simulink model "ChiefMaster_TTC580"  (R2022b)
settings: Solver=FixedStepAuto  StartTime=0.0  StopTime=10  FixedStep=0.01  RelTol=1e-3
values from neighbouring files (symbols this model uses):
  BattBox1_No = single(1)    [Parameters.m]
  BattBox2_No = single(2)    [Parameters.m]
  BattBox3_No = single(3)    [Parameters.m]
  CurrentLB = single(-3)    [Parameters.m]
  CurrentReductionConstant_Lvl0 = single(0.03)    [Parameters.m]
  CurrentReductionConstant_Lvl1 = single(0.05)    [Parameters.m]
  CurrentReductionConstant_Lvl2 = single(0.07)    [Parameters.m]
  CurrentReductionConstant_Lvl3 = single(0.1)    [Parameters.m]
  CurrentUB = single(3)    [Parameters.m]
  DCHV_Minus_In_Delay_ms = single(500)    [Parameters.m]
  FL_sHVC_CellBalanceVoltage_mV = single(3500)    [Parameters.m]
  FL_sInrushCurrent_dividebyzero = single(0.00001)    [Parameters.m]
  FL_u8HMI_BuzzerTimer = uint8(3)    [Parameters.m]
  IP_boActValue = true    [Parameters.m]
  IP_boDeactValue = false    [Parameters.m]
  IP_boInitValue = false    [Parameters.m]
  IP_s_LB = 18000    [Parameters.m]
  IP_s_UB = 22000    [Parameters.m]
  IP_sBatt1_ChargeCurrentMax_Factor = single(0.1)    [Parameters.m]
  IP_sBatt1_ChargeCurrentMax_LB = single(0)    [Parameters.m]
  IP_sBatt1_ChargeCurrentMax_Offset = single(0)    [Parameters.m]
  IP_sBatt1_ChargeCurrentMax_UB = single(6553.5)    [Parameters.m]
  IP_sBatt1_Current_Factor = single(0.1)    [Parameters.m]
  IP_sBatt1_Current_LB = single(-3276.8)    [Parameters.m]
  IP_sBatt1_Current_Offset = single(0)    [Parameters.m]
  IP_sBatt1_Current_UB = single(3276.8)    [Parameters.m]
  IP_sBatt1_DisChargeCurrentMax_Factor = single(0.1)    [Parameters.m]
  IP_sBatt1_DisChargeCurrentMax_LB = single(0)    [Parameters.m]
  IP_sBatt1_DisChargeCurrentMax_Offset = single(0)    [Parameters.m]
  IP_sBatt1_DisChargeCurrentMax_UB = single(6553.5)    [Parameters.m]
  IP_sBatt1_InsulationResistance_Factor = single(5)    [Parameters.m]
  IP_sBatt1_InsulationResistance_LB = single(0)    [Parameters.m]
  IP_sBatt1_InsulationResistance_Offset = single(0)    [Parameters.m]
  IP_sBatt1_InsulationResistance_UB = single(0)    [Parameters.m]
  IP_sBatt1_LiBa_IntResist_mOhm = single(25)    [Parameters.m]
  IP_sBatt1_SOC_Factor = single(1)    [Parameters.m]
  IP_sBatt1_SOC_LB = single(0)    [Parameters.m]
  IP_sBatt1_SOC_Offset = single(0)    [Parameters.m]
  IP_sBatt1_SOC_UB = single(100)    [Parameters.m]
  IP_sBatt1_SOH_Factor = single(1)    [Parameters.m]
  IP_sBatt1_SOH_LB = single(0)    [Parameters.m]
  IP_sBatt1_SOH_Offset = single(0)    [Parameters.m]
  IP_sBatt1_SOH_UB = single(100)    [Parameters.m]
  IP_sBatt1_Ubatt_Factor = single(0.1)    [Parameters.m]
  IP_sBatt1_Ubatt_LB = single(0)    [Parameters.m]
  IP_sBatt1_Ubatt_Offset = single(0)    [Parameters.m]
  IP_sBatt1_Ubatt_UB = single(6553.5)    [Parameters.m]
  IP_sBatt1_UserRi_Factor = single(1)    [Parameters.m]
  IP_sBatt1_UserRi_LB = single(0)    [Parameters.m]
  IP_sBatt1_UserRi_Offset = single(0)    [Parameters.m]
  IP_sBatt1_UserRi_UB = single(255)    [Parameters.m]
  IP_sBatt1_VoltageAtSensor_Factor = single(0.02)    [Parameters.m]
  IP_sBatt1_VoltageAtSensor_LB = single(0)    [Parameters.m]
  IP_sBatt1_VoltageAtSensor_Offset = single(0)    [Parameters.m]
  IP_sBatt1_VoltageAtSensor_UB = single(1310.7)    [Parameters.m]
  IP_sBatt2_LiBa_IntResist_mOhm = single(25)    [Parameters.m]
  IP_sBatt3_LiBa_IntResist_mOhm = single(25)    [Parameters.m]
  IP_sEM_LB = 2000    [Parameters.m]
  IP_sEM_UB = 8000    [Parameters.m]
  IP_sFB_LB = 5000    [Parameters.m]
  IP_sFB_UB = 10000    [Parameters.m]
  IP_sHVIL_LB = 12000    [Parameters.m]
  IP_sHVIL_UB = 15000    [Parameters.m]
  IP_sLoad_Voltage_Factor = single(1)    [Parameters.m]
  IP_sLoad_Voltage_LB = single(0)    [Parameters.m]
  IP_sLoad_Voltage_Offset = single(0)    [Parameters.m]
  IP_sLoad_Voltage_UB = single(65535)    [Parameters.m]
  IP_u8HVIL_Delay_ms = uint8(100)    [Parameters.m]
  IP_u8HW_IN_delay_ms = uint8(100)    [Parameters.m]
  IT_sInsulationSafeValue_kOhm = single(650)    [Parameters.m]
  IT_u8IMD_DelayTime_s = uint8(20)    [Parameters.m]
  MainHV_Minus_In_Delay = single(5)    [Parameters.m]
  MainHV_StatusDelay = single(5)    [Parameters.m]
  NotAvailable_uint16 = single(65535)    [Parameters.m]
  NotAvailable_uint8 = uint8(255)    [Parameters.m]
  OP_boHVIL_Supply = boolean(1)    [Parameters.m]
  SafeCurrentToCloseHV_A = single(5)    [Parameters.m]
  SafeVoltageToCloseHV_V = single(0.5)    [Parameters.m]
  UnexpectedBattChargingFcn_Available = boolean(1)    [Parameters.m]
  Voltage_NA_UB = uint16(65535)    [Parameters.m]
  VoltageSensorAvailableBB1 = boolean(0)    [Parameters.m]
  VoltageSensorAvailableBB2 = boolean(0)    [Parameters.m]
  VoltageSensorAvailableBB3 = boolean(0)    [Parameters.m]
libraries: simulink x184, Library_DataProcessing_v1_1 x167, Library_DataProcessing_v1 x142, libCM x28
(part 8 of 19)

== system ChiefMaster_TTC580/ChiefMaster/Input Translation/Battery Signals/Subsystem9 ==
  IP_Databus : Inport
  Bus Selector1 : BusSelector  OutputSignals=IP_Actia_BatBox_DataBus.IP_Actia_Batt1_Databus.Batt1_MyStatus2_Databus.IP_boBatt1_HV_relay_MINUS_Sense,IP_LB_BattBox_DataBus.IP_LB_BattBox1_DataBus.IP_LB_Batt1_Status01_DataBus.IP_LB_BMS_IO_state_Input_DataBus,IP_Actia_BatBox_DataBus.IP_Actia_Batt1_Databus.Batt1_MyStatus2_Databus.IP_boBatt1_HV_relay_PLUS_Sense,IP_Actia_BatBox_DataBus.IP_Actia_Batt2_Databus.Batt2_MyStatus2_Databus.IP_boBatt2_HV_relay_MINUS_Sense,IP_LB_BattBox_DataBus.IP_LB_BattBox2_DataBus.IP_LB_Batt2_Status01_DataBus.IP_LB_BMS_IO_state_Input_DataBus,IP_Actia_BatBox_DataBus.IP_Actia_Batt2_Databus.Batt2_MyStatus2_Databus.IP_boBatt2_HV_relay_PLUS_Sense,IP_Actia_BatBox_DataBus.IP_Actia_Batt3_Databus.Batt3_MyStatus2_Databus.IP_boBatt3_HV_relay_MINUS_Sense,IP_LB_BattBox_DataBus.IP_LB_BattBox3_DataBus.IP_LB_Batt3_Status01_DataBus.IP_LB_BMS_IO_state_Input_DataBus,IP_Actia_BatBox_DataBus.IP_Actia_Batt3_Databus.Batt3_MyStatus2_Databus.IP_boBatt3_HV_relay_PLUS_Sense
  Subsystem1 : Subsystem
  Subsystem2 : Subsystem
  Subsystem3 : Subsystem
  Subsystem4 : Subsystem
  Subsystem5 : Subsystem
  Subsystem8 : Subsystem
  IP_boBMS_HV_Minus_Sense_BB1 : Outport
  IP_boBMS_HV_Plus_Sense_BB1 : Outport  Port=2
  IP_boBMS_HV_Minus_Sense_BB2 : Outport  Port=3
  IP_boBMS_HV_Plus_Sense_BB2 : Outport  Port=4
  IP_boBMS_HV_Minus_Sense_BB3 : Outport  Port=5
  IP_boBMS_HV_Plus_Sense_BB3 : Outport  Port=6
  wires:
  Bus Selector1/6 -> Subsystem2/2(<IP_boBatt1_HV_relay_PLUS_Sense>)  "<IP_boBatt2_HV_relay_PLUS_Sense>"
  Bus Selector1/2 -> Subsystem8/2(<IP_LB_BMS_IO_state_Input_DataBus>), Subsystem1/1(<IP_LB_BMS_IO_state_Input_DataBus>)  "<IP_LB_BMS_IO_state_Input_DataBus>"
  Bus Selector1/5 -> Subsystem3/2(<IP_LB_BMS_IO_state_Input_DataBus>), Subsystem2/1(<IP_LB_BMS_IO_state_Input_DataBus>)  "<IP_LB_BMS_IO_state_Input_DataBus>"
  Bus Selector1/7 -> Subsystem5/1(<IP_boBatt3_HV_relay_MINUS_Sense>)  "<IP_boBatt3_HV_relay_MINUS_Sense>"
  Bus Selector1/9 -> Subsystem4/2(<IP_boBatt3_HV_relay_PLUS_Sense>)  "<IP_boBatt3_HV_relay_PLUS_Sense>"
  Bus Selector1/8 -> Subsystem5/2(<IP_LB_BMS_IO_state_Input_DataBus>), Subsystem4/1(<IP_LB_BMS_IO_state_Input_DataBus>)  "<IP_LB_BMS_IO_state_Input_DataBus>"
  Subsystem8/1(IP_boBMS_HV_Minus_Sense_BB1) -> IP_boBMS_HV_Minus_Sense_BB1/1
  IP_Databus/1 -> Bus Selector1/1
  Subsystem1/1(IP_boBMS_HV_Plus_Sense_BB1) -> IP_boBMS_HV_Plus_Sense_BB1/1
  Bus Selector1/4 -> Subsystem3/1(<IP_boBatt2_HV_relay_MINUS_Sense>)  "<IP_boBatt2_HV_relay_MINUS_Sense>"
  Subsystem2/1(IP_boBMS_HV_Plus_Sense_BB2) -> IP_boBMS_HV_Plus_Sense_BB2/1
  Subsystem3/1(IP_boBMS_HV_Minus_Sense_BB2) -> IP_boBMS_HV_Minus_Sense_BB2/1
  Subsystem5/1(IP_boBMS_HV_Minus_Sense_BB3) -> IP_boBMS_HV_Minus_Sense_BB3/1
  Subsystem4/1(IP_boBMS_HV_Plus_Sense_BB3) -> IP_boBMS_HV_Plus_Sense_BB3/1
  Bus Selector1/3 -> Subsystem1/2(<IP_boBatt1_HV_relay_PLUS_Sense>)  "<IP_boBatt1_HV_relay_PLUS_Sense>"
  Bus Selector1/1 -> Subsystem8/1(<IP_boBatt1_HV_relay_MINUS_Sense>)  "<IP_boBatt1_HV_relay_MINUS_Sense>"

== system ChiefMaster_TTC580/ChiefMaster/Output Processing/CM_OBD/CM_BDU_Msg5_6 ==
  OT_Databus : Inport
  Bus Selector1 : BusSelector  OutputSignals=OT_BDUControl_Databus.OT_boREQ_MainHV_ON_MINUS,OT_BDUControl_Databus.OT_boREQ_MainHV_ON_Precharge,OT_BDUControl_Databus.OT_boREQ_MainHV_ON_PLUS,OT_BDUControl_Databus.OT_boMainHV_Minus_Welded,OT_BDUControl_Databus.OT_boMainHV_Plus_Welded,OT_BDUControl_Databus.OT_boMainHV_WeldingCheckActive,OT_BDUControl_Databus.OT_u8MainHV_Minus_Status,OT_BDUControl_Databus.OT_u8MainHV_Plus_Status,OT_BDUControl_Databus.OT_u8Precharge_Status,OT_BDUControl_Databus.OT_u8WeldingDetection_Status,OT_BDUControl_Databus.OT_u8DCHV_Minus_Status,OT_BDUControl_Databus.OT_u8DCHV_plus_Status
  Bus Selector9 : BusSelector  OutputSignals=FL_Databus.FL_BatteryBox_HVControl_Databus.FL_sCalculated_VoltageDiff_BB1,FL_Databus.FL_BatteryBox_HVControl_Databus.FL_sCalculated_VoltageDiff_BB2,FL_Databus.FL_BatteryBox_HVControl_Databus.FL_sCalculated_VoltageDiff_BB3,FL_Databus.FL_BatteryBox_HVControl_Databus.FL_sCalculated_InrushCurrent_BB1,FL_Databus.FL_BatteryBox_HVControl_Databus.FL_sCalculated_InrushCurrent_BB2,FL_Databus.FL_BatteryBox_HVControl_Databus.FL_sCalculated_InrushCurrent_BB3
  Constant : Constant  Value=0  OutDataTypeStr=uint8
  Constant1 : Constant  Value=0  OutDataTypeStr=uint8
  Constant2 : Constant  Value=0  OutDataTypeStr=uint8
  Extract Bits{1..6} (6 alike) : simulink/Logic and Bit Operations/Extract Bits  bitsToExtract=Range of bits  numBits=8  bitIdxRange=[0 1]  outScalingMode=Preserve fixed-point scaling
  Lib_MultiBit_Concat1 : Library_DataProcessing_v1/Lib_MultiBit_Concat  SystemSampleTime=-1  VariantActivationTime=update diagram  Latency=0  AutoFrameSizeCalculation=off
  Lib_MultiBit_Concat2 : Library_DataProcessing_v1/Lib_MultiBit_Concat  SystemSampleTime=-1  VariantActivationTime=update diagram  Latency=0  AutoFrameSizeCalculation=off
  Lib_MultiBit_Concat7 : Library_DataProcessing_v1/Lib_MultiBit_Concat  SystemSampleTime=-1  VariantActivationTime=update diagram  Latency=0  AutoFrameSizeCalculation=off
  Mux3 : Mux  Inputs=8
  Mux4 : Mux  Inputs=8
  Subsystem1 : Subsystem
  Subsystem4 : Subsystem
  Subsystem5 : Subsystem
  Subsystem6 : Subsystem
  Subsystem8 : Subsystem
  Subsystem9 : Subsystem
  "Chief_Master_Calc_Msg5 " : Outport
  Chief_Master_BDU_Msg6 : Outport  Port=2
  wires:
  Extract Bits4/1 -> Lib_MultiBit_Concat1/5
  Bus Selector1/3 -> Lib_MultiBit_Concat7/3  "<OT_boREQ_MainHV_ON_PLUS>"
  Lib_MultiBit_Concat1/1 -> Mux4/6
  Constant/1 -> Lib_MultiBit_Concat1/8, Lib_MultiBit_Concat1/2, Lib_MultiBit_Concat7/8, Lib_MultiBit_Concat1/4, Lib_MultiBit_Concat1/6, Lib_MultiBit_Concat1/7
  Bus Selector9/1 -> Subsystem4/1(Calculated_VtgDiff_BB1)  "<FL_sCalculated_VoltageDiff_BB1>"
  Extract Bits2/1 -> Lib_MultiBit_Concat7/7
  Subsystem4/2(u8byte_MSB) -> Mux3/2
  Subsystem6/2(u8byte_MSB) -> Mux3/6
  Bus Selector1/5 -> Lib_MultiBit_Concat7/5  "<OT_boMainHV_Plus_Welded>"
  Bus Selector1/10 -> Extract Bits4/1  "<OT_u8WeldingDetection_Status>"
  Bus Selector1/8 -> Extract Bits1/1  "<OT_u8MainHV_Plus_Status>"
  Extract Bits3/1 -> Lib_MultiBit_Concat1/3
  Subsystem5/2(u8byte_MSB) -> Mux3/4
  Lib_MultiBit_Concat7/1 -> Mux4/5
  Subsystem4/1(u8byte_LSB) -> Mux3/1
  Subsystem9/2(u8byte_MSB) -> Mux4/4
  Subsystem1/1(u8byte_LSB) -> Mux3/7
  Subsystem5/1(u8byte_LSB) -> Mux3/3
  Subsystem9/1(u8byte_LSB) -> Mux4/3
  Subsystem6/1(u8byte_LSB) -> Mux3/5
  Bus Selector9/2 -> Subsystem5/1(Calculated_VtgDiff_BB2)  "<FL_sCalculated_VoltageDiff_BB2>"
  Bus Selector9/5 -> Subsystem8/1(Calculated_InrushCurr_BB2)  "<FL_sCalculated_InrushCurrent_BB2>"
  Bus Selector9/3 -> Subsystem6/1(Calculated_VtgDiff_BB3)  "<FL_sCalculated_VoltageDiff_BB3>"
  Bus Selector1/4 -> Lib_MultiBit_Concat7/4  "<OT_boMainHV_Minus_Welded>"
  Bus Selector9/4 -> Subsystem1/1(Calculated_InrushCurr_BB2)  "<FL_sCalculated_InrushCurrent_BB1>"
  Bus Selector9/6 -> Subsystem9/1(Calculated_InrushCurr_BB3)  "<FL_sCalculated_InrushCurrent_BB3>"
  Bus Selector1/7 -> Extract Bits2/1  "<OT_u8MainHV_Minus_Status>"
  Bus Selector1/1 -> Lib_MultiBit_Concat7/1  "<OT_boREQ_MainHV_ON_MINUS>"
  Subsystem8/2(u8byte_MSB) -> Mux4/2
  Bus Selector1/9 -> Extract Bits3/1  "<OT_u8Precharge_Status>"
  Constant1/1 -> Mux4/8
  Mux4/1 -> Chief_Master_BDU_Msg6/1
  Mux3/1 -> "Chief_Master_Calc_Msg5 "/1
  Subsystem8/1(u8byte_LSB) -> Mux4/1
  Bus Selector1/2 -> Lib_MultiBit_Concat7/2  "<OT_boREQ_MainHV_ON_Precharge>"
  OT_Databus/1 -> Bus Selector1/1, Bus Selector9/1
  Subsystem1/2(u8byte_MSB) -> Mux3/8
  Bus Selector1/6 -> Lib_MultiBit_Concat7/6  "<OT_boMainHV_WeldingCheckActive>"
  Extract Bits1/1 -> Lib_MultiBit_Concat1/1
  Constant2/1 -> Lib_MultiBit_Concat2/8, Lib_MultiBit_Concat2/7, Lib_MultiBit_Concat2/6, Lib_MultiBit_Concat2/5, Lib_MultiBit_Concat2/4, Lib_MultiBit_Concat2/2
  Lib_MultiBit_Concat2/1 -> Mux4/7
  Bus Selector1/11 -> Extract Bits5/1  "<OT_u8DCHV_Minus_Status>"
  Extract Bits5/1 -> Lib_MultiBit_Concat2/1
  Extract Bits6/1 -> Lib_MultiBit_Concat2/3
  Bus Selector1/12 -> Extract Bits6/1  "<OT_u8DCHV_plus_Status>"

== system ChiefMaster_TTC580/ChiefMaster/Output Processing/CM_OBD/CM_Battery1_Msg7 ==
  OT_Databus : Inport
  Bus Selector1 : BusSelector  OutputSignals=FL_Databus.IT_Databus.IT_BatterySignal_Databus.IT_sBMS_VtgInt_BB1,FL_Databus.IT_Databus.IT_BatterySignal_Databus.IT_sBMS_Current_BB1,FL_Databus.IT_Databus.IT_BatterySignal_Databus.IT_u8BMS_SOC_BB1,FL_Databus.IT_Databus.IT_BatterySignal_Databus.IT_sBMS_InternalResistance_BB1_ohms
  Bus Selector2 : BusSelector  OutputSignals=FL_Databus.IT_Databus.IT_BatterySignal_Databus.IT_boBMS_HV_REL_ON_BB1,FL_Databus.IT_Databus.IT_BatterySignal_Databus.IT_boBMS_HV_Minus_Sense_BB1,FL_Databus.IT_Databus.IT_BatterySignal_Databus.IT_boBMS_HV_Plus_Sense_BB1,FL_Databus.IT_Databus.IT_BatterySignal_Databus.IT_boBMS_InsulationReadyOK_B1,FL_Databus.IT_Databus.IT_BatterySignal_Databus.IT_boBMS_InsulationSDError_B1,FL_Databus.IT_Databus.IT_BatterySignal_Databus.IT_boBMS_IMD_Active_BB1,FL_Databus.IT_Databus.IT_BatterySignal_Databus.IT_boBMS_Error_BB1,FL_Databus.IT_Databus.IT_BatterySignal_Databus.IT_boBMS_Warning_BB1
  Bus Selector6 : BusSelector  OutputSignals=FL_Databus.IT_Databus.IT_BatterySignal_Databus.IT_boBMS_Batt1_Availability,OT_IMD_Databus.OT_boREQ_IMD_ON_BB1,OT_BatteryBox_HVControl_Databus.OT_u8ContactorState_BB1,OT_BatteryBox_HVControl_Databus.OT_boREQ_HV_ON_BB1,OT_BatteryBox_HVControl_Databus.OT_u8Contactor_FB_State_BB1,FL_Databus.IT_Databus.IT_BatterySignal_Databus.IT_boBMS_SDError_BB1
  Constant : Constant  Value=0  OutDataTypeStr=single
  Constant1 : Constant  Value=0  OutDataTypeStr=single
  Constant2 : Constant  Value=0.1  OutDataTypeStr=single
  Constant3 : Constant  Value=0.1  OutDataTypeStr=single
  Constant4 : Constant  Value=0  OutDataTypeStr=uint8
  Data Type Conversion1 : DataTypeConversion  OutDataTypeStr=uint8  SaturateOnIntegerOverflow=off  RndMeth=Floor
  Extract Bits1 : simulink/Logic and Bit Operations/Extract Bits  bitsToExtract=Range of bits  numBits=8  bitIdxRange=[0 1]  outScalingMode=Preserve fixed-point scaling
  Extract Bits2 : simulink/Logic and Bit Operations/Extract Bits  bitsToExtract=Range of bits  numBits=8  bitIdxRange=[0 1]  outScalingMode=Preserve fixed-point scaling
  Lib_2bytes_Split1 : Library_DataProcessing_v1/Lib_2bytes_Split  SystemSampleTime=-1  VariantActivationTime=update diagram  Latency=0  AutoFrameSizeCalculation=off
  Lib_2bytes_Split2 : Library_DataProcessing_v1/Lib_2bytes_Split  SystemSampleTime=-1  VariantActivationTime=update diagram  Latency=0  AutoFrameSizeCalculation=off
  Lib_MultiBit_Concat1 : Library_DataProcessing_v1/Lib_MultiBit_Concat  SystemSampleTime=-1  VariantActivationTime=update diagram  Latency=0  AutoFrameSizeCalculation=off
  Lib_MultiBit_Concat2 : Library_DataProcessing_v1/Lib_MultiBit_Concat  SystemSampleTime=-1  VariantActivationTime=update diagram  Latency=0  AutoFrameSizeCalculation=off
  Lib_OutProcessing1 : Library_DataProcessing_v1/Lib_OutProcessing  SystemSampleTime=-1  VariantActivationTime=update diagram  Latency=0  AutoFrameSizeCalculation=off
  Lib_OutProcessing2 : Library_DataProcessing_v1/Lib_OutProcessing  SystemSampleTime=-1  VariantActivationTime=update diagram  Latency=0  AutoFrameSizeCalculation=off
  Mux : Mux  Inputs=8
  OP_ChiefMaster_Battery1_Msg7 : Outport
  wires:
  Mux/1 -> OP_ChiefMaster_Battery1_Msg7/1
  OT_Databus/1 -> Bus Selector1/1, Bus Selector2/1, Bus Selector6/1
  Bus Selector6/1 -> Lib_MultiBit_Concat1/1  "<IT_boBMS_Batt1_Availability>"
  Bus Selector6/2 -> Lib_MultiBit_Concat1/2  "<OT_boREQ_IMD_ON_BB1>"
  Bus Selector6/3 -> Extract Bits2/1  "<OT_u8ContactorState_BB1>"
  Bus Selector6/4 -> Lib_MultiBit_Concat1/5  "<OT_boREQ_HV_ON_BB1>"
  Bus Selector6/5 -> Extract Bits1/1  "<OT_u8Contactor_FB_State_BB1>"
  Lib_MultiBit_Concat1/1 -> Mux/1
  Lib_MultiBit_Concat2/1 -> Mux/2
  Constant/1 -> Lib_OutProcessing1/2
  Constant2/1 -> Lib_OutProcessing1/3
  Lib_OutProcessing1/1 -> Lib_2bytes_Split1/1
  Bus Selector1/1 -> Lib_OutProcessing1/1  "<IT_sBMS_VtgInt_BB1>"
  Lib_2bytes_Split1/1 -> Mux/3
  Lib_2bytes_Split1/2 -> Mux/4
  Bus Selector1/2 -> Lib_OutProcessing2/1  "<IT_sBMS_Current_BB1>"
  Lib_OutProcessing2/1 -> Lib_2bytes_Split2/1
  Constant3/1 -> Lib_OutProcessing2/3
  Constant1/1 -> Lib_OutProcessing2/2
  Lib_2bytes_Split2/1 -> Mux/5
  Lib_2bytes_Split2/2 -> Mux/6
  Bus Selector1/3 -> Mux/7  "<IT_u8BMS_SOC_BB1>"
  Bus Selector1/4 -> Data Type Conversion1/1  "<IT_sBMS_InternalResistance_BB1_ohms>"
  Data Type Conversion1/1 -> Mux/8
  Constant4/1 -> Lib_MultiBit_Concat1/4, Lib_MultiBit_Concat1/7
  Extract Bits2/1 -> Lib_MultiBit_Concat1/3
  Extract Bits1/1 -> Lib_MultiBit_Concat1/6
  Bus Selector6/6 -> Lib_MultiBit_Concat1/8  "<IT_boBMS_SDError_BB1>"
  Bus Selector2/1 -> Lib_MultiBit_Concat2/1  "<IT_boBMS_HV_REL_ON_BB1>"
  Bus Selector2/2 -> Lib_MultiBit_Concat2/2  "<IT_boBMS_HV_Minus_Sense_BB1>"
  Bus Selector2/3 -> Lib_MultiBit_Concat2/3  "<IT_boBMS_HV_Plus_Sense_BB1>"
  Bus Selector2/4 -> Lib_MultiBit_Concat2/4  "<IT_boBMS_InsulationReadyOK_B1>"
  Bus Selector2/5 -> Lib_MultiBit_Concat2/5  "<IT_boBMS_InsulationSDError_B1>"
  Bus Selector2/6 -> Lib_MultiBit_Concat2/6  "<IT_boBMS_IMD_Active_BB1>"
  Bus Selector2/7 -> Lib_MultiBit_Concat2/7  "<IT_boBMS_Error_BB1>"
  Bus Selector2/8 -> Lib_MultiBit_Concat2/8  "<IT_boBMS_Warning_BB1>"

== system ChiefMaster_TTC580/ChiefMaster/Output Processing/CM_OBD/CM_Battery1_Msg8 ==
  OT_Databus : Inport
  Bus Selector1 : BusSelector  OutputSignals=FL_Databus.IT_Databus.IT_BatterySignal_Databus.IT_sBMS_ChargeCurrentPrognosis_BB1,FL_Databus.IT_Databus.IT_BatterySignal_Databus.IT_sBMS_DisChargeCurrentPrognosis_BB1,FL_Databus.IT_Databus.IT_BatterySignal_Databus.IT_sBMS_InsulationResistance_BB1,FL_Databus.IT_Databus.IT_BatterySignal_Databus.IT_boBMS_InsulationResistance_Minus_kOhm_BB1
  Constant{1..2,5,7} (4 alike) : Constant  Value=0  OutDataTypeStr=single
  Constant3 : Constant  Value=0.1  OutDataTypeStr=single
  Constant4 : Constant  Value=0.1  OutDataTypeStr=single
  Constant6 : Constant  Value=100  OutDataTypeStr=single
  Constant8 : Constant  Value=100  OutDataTypeStr=single
  Lib_2bytes_Split{1..4} (4 alike) : Library_DataProcessing_v1/Lib_2bytes_Split  SystemSampleTime=-1  VariantActivationTime=update diagram  Latency=0  AutoFrameSizeCalculation=off
  Lib_OutProcessing{1..4} (4 alike) : Library_DataProcessing_v1/Lib_OutProcessing  SystemSampleTime=-1  VariantActivationTime=update diagram  Latency=0  AutoFrameSizeCalculation=off
  Mux : Mux  Inputs=8
  OP_ChiefMaster_Battery1_Msg8 : Outport
  wires:
  OT_Databus/1 -> Bus Selector1/1
  Mux/1 -> OP_ChiefMaster_Battery1_Msg8/1
  Bus Selector1/1 -> Lib_OutProcessing2/1  "<IT_sBMS_ChargeCurrentPrognosis_BB1>"
  Bus Selector1/2 -> Lib_OutProcessing1/1  "<IT_sBMS_DisChargeCurrentPrognosis_BB1>"
  Bus Selector1/3 -> Lib_OutProcessing3/1  "<IT_sBMS_InsulationResistance_BB1>"
  Bus Selector1/4 -> Lib_OutProcessing4/1  "<IT_boBMS_InsulationResistance_Minus_kOhm_BB1>"
  Constant3/1 -> Lib_OutProcessing2/3
  Lib_OutProcessing2/1 -> Lib_2bytes_Split2/1
  Constant1/1 -> Lib_OutProcessing2/2
  Lib_2bytes_Split2/1 -> Mux/1
  Lib_2bytes_Split2/2 -> Mux/2
  Constant2/1 -> Lib_OutProcessing1/2
  Lib_OutProcessing1/1 -> Lib_2bytes_Split1/1
  Constant4/1 -> Lib_OutProcessing1/3
  Lib_2bytes_Split1/1 -> Mux/3
  Lib_2bytes_Split1/2 -> Mux/4
  Constant6/1 -> Lib_OutProcessing3/3
  Lib_OutProcessing3/1 -> Lib_2bytes_Split3/1
  Constant5/1 -> Lib_OutProcessing3/2
  Lib_2bytes_Split3/1 -> Mux/5
  Lib_2bytes_Split3/2 -> Mux/6
  Constant7/1 -> Lib_OutProcessing4/2
  Lib_OutProcessing4/1 -> Lib_2bytes_Split4/1
  Constant8/1 -> Lib_OutProcessing4/3
  Lib_2bytes_Split4/1 -> Mux/7
  Lib_2bytes_Split4/2 -> Mux/8

== system ChiefMaster_TTC580/ChiefMaster/Output Processing/CM_OBD/CM_Battery1_Msg9 ==
  OT_Databus : Inport
  Bus Selector1 : BusSelector  OutputSignals=FL_Databus.IT_Databus.IT_BatterySignal_Databus.IP_sBMS_MinTemp_degC_BB1,FL_Databus.IT_Databus.IT_BatterySignal_Databus.IP_sBMS_MaxTemp_degC_BB1,FL_Databus.IT_Databus.IT_BatterySignal_Databus.IP_sBMS_MinCellVoltage_BB1,FL_Databus.IT_Databus.IT_BatterySignal_Databus.IP_sBMS_MaxCellVoltage_BB1
  Constant1 : Constant  Value=-40  OutDataTypeStr=single
  Constant2 : Constant  Value=-40  OutDataTypeStr=single
  Constant3 : Constant  OutDataTypeStr=single
  Constant4 : Constant  OutDataTypeStr=single
  Constant5 : Constant  Value=0  OutDataTypeStr=single
  Constant6 : Constant  Value=0.1  OutDataTypeStr=single
  Constant7 : Constant  Value=0  OutDataTypeStr=single
  Constant8 : Constant  Value=0.1  OutDataTypeStr=single
  Constant9 : Constant  Value=0  OutDataTypeStr=uint8
  Data Type Conversion : DataTypeConversion  OutDataTypeStr=uint8  SaturateOnIntegerOverflow=off  RndMeth=Floor
  Data Type Conversion1 : DataTypeConversion  OutDataTypeStr=uint8  SaturateOnIntegerOverflow=off  RndMeth=Floor
  Lib_2bytes_Split3 : Library_DataProcessing_v1/Lib_2bytes_Split  SystemSampleTime=-1  VariantActivationTime=update diagram  Latency=0  AutoFrameSizeCalculation=off
  Lib_2bytes_Split4 : Library_DataProcessing_v1/Lib_2bytes_Split  SystemSampleTime=-1  VariantActivationTime=update diagram  Latency=0  AutoFrameSizeCalculation=off
  Lib_OutProcessing{1..4} (4 alike) : Library_DataProcessing_v1/Lib_OutProcessing  SystemSampleTime=-1  VariantActivationTime=update diagram  Latency=0  AutoFrameSizeCalculation=off
  Mux : Mux  Inputs=8
  OP_ChiefMaster_Battery1_Msg8 : Outport
  wires:
  Constant8/1 -> Lib_OutProcessing4/3
  Lib_OutProcessing4/1 -> Lib_2bytes_Split4/1
  Constant7/1 -> Lib_OutProcessing4/2
  Constant5/1 -> Lib_OutProcessing3/2
  Lib_OutProcessing3/1 -> Lib_2bytes_Split3/1
  Constant6/1 -> Lib_OutProcessing3/3
  Constant4/1 -> Lib_OutProcessing1/3
  Lib_OutProcessing1/1 -> Data Type Conversion1/1
  Constant2/1 -> Lib_OutProcessing1/2
  Constant1/1 -> Lib_OutProcessing2/2
  Lib_OutProcessing2/1 -> Data Type Conversion/1
  Constant3/1 -> Lib_OutProcessing2/3
  Bus Selector1/4 -> Lib_OutProcessing4/1  "<IP_sBMS_MaxCellVoltage_BB1>"
  Bus Selector1/3 -> Lib_OutProcessing3/1  "<IP_sBMS_MinCellVoltage_BB1>"
  Bus Selector1/2 -> Lib_OutProcessing1/1  "<IP_sBMS_MaxTemp_degC_BB1>"
  Bus Selector1/1 -> Lib_OutProcessing2/1  "<IP_sBMS_MinTemp_degC_BB1>"
  Mux/1 -> OP_ChiefMaster_Battery1_Msg8/1
  OT_Databus/1 -> Bus Selector1/1
  Constant9/1 -> Mux/7, Mux/8
  Lib_2bytes_Split3/1 -> Mux/3
  Lib_2bytes_Split3/2 -> Mux/4
  Lib_2bytes_Split4/1 -> Mux/5
  Lib_2bytes_Split4/2 -> Mux/6
  Data Type Conversion/1 -> Mux/1
  Data Type Conversion1/1 -> Mux/2

== system ChiefMaster_TTC580/ChiefMaster/Output Processing/CM_OBD/CM_Battery2_Msg10 ==
  OT_Databus : Inport
  Bus Selector1 : BusSelector  OutputSignals=FL_Databus.IT_Databus.IT_BatterySignal_Databus.IT_sBMS_VtgInt_BB2,FL_Databus.IT_Databus.IT_BatterySignal_Databus.IT_sBMS_Current_BB2,FL_Databus.IT_Databus.IT_BatterySignal_Databus.IT_u8BMS_SOC_BB2,FL_Databus.IT_Databus.IT_BatterySignal_Databus.IT_sBMS_InternalResistance_BB2_ohms
  Bus Selector2 : BusSelector  OutputSignals=FL_Databus.IT_Databus.IT_BatterySignal_Databus.IT_boBMS_HV_REL_ON_BB2,FL_Databus.IT_Databus.IT_BatterySignal_Databus.IT_boBMS_HV_Minus_Sense_BB2,FL_Databus.IT_Databus.IT_BatterySignal_Databus.IT_boBMS_HV_Plus_Sense_BB2,FL_Databus.IT_Databus.IT_BatterySignal_Databus.IT_boBMS_InsulationReadyOK_B2,FL_Databus.IT_Databus.IT_BatterySignal_Databus.IT_boBMS_InsulationSDError_B2,FL_Databus.IT_Databus.IT_BatterySignal_Databus.IT_boBMS_IMD_Active_BB2,FL_Databus.IT_Databus.IT_BatterySignal_Databus.IT_boBMS_Error_BB2,FL_Databus.IT_Databus.IT_BatterySignal_Databus.IT_boBMS_Warning_BB2
  Bus Selector6 : BusSelector  OutputSignals=FL_Databus.IT_Databus.IT_BatterySignal_Databus.IT_boBMS_Batt2_Availability,OT_IMD_Databus.OT_boREQ_IMD_ON_BB2,OT_BatteryBox_HVControl_Databus.OT_u8ContactorState_BB2,OT_BatteryBox_HVControl_Databus.OT_boREQ_HV_ON_BB2,OT_BatteryBox_HVControl_Databus.OT_u8Contactor_FB_State_BB2,FL_Databus.IT_Databus.IT_BatterySignal_Databus.IT_boBMS_SDError_BB2
  Constant : Constant  Value=0  OutDataTypeStr=single
  Constant1 : Constant  Value=0  OutDataTypeStr=single
  Constant2 : Constant  Value=0.1  OutDataTypeStr=single
  Constant3 : Constant  Value=0.1  OutDataTypeStr=single
  Constant4 : Constant  Value=0  OutDataTypeStr=uint8
  Data Type Conversion : DataTypeConversion  SaturateOnIntegerOverflow=off  RndMeth=Floor
  Extract Bits1 : simulink/Logic and Bit Operations/Extract Bits  bitsToExtract=Range of bits  numBits=8  bitIdxRange=[0 1]  outScalingMode=Preserve fixed-point scaling
  Extract Bits2 : simulink/Logic and Bit Operations/Extract Bits  bitsToExtract=Range of bits  numBits=8  bitIdxRange=[0 1]  outScalingMode=Preserve fixed-point scaling
  Lib_2bytes_Split1 : Library_DataProcessing_v1/Lib_2bytes_Split  SystemSampleTime=-1  VariantActivationTime=update diagram  Latency=0  AutoFrameSizeCalculation=off
  Lib_2bytes_Split2 : Library_DataProcessing_v1/Lib_2bytes_Split  SystemSampleTime=-1  VariantActivationTime=update diagram  Latency=0  AutoFrameSizeCalculation=off
  Lib_MultiBit_Concat1 : Library_DataProcessing_v1/Lib_MultiBit_Concat  SystemSampleTime=-1  VariantActivationTime=update diagram  Latency=0  AutoFrameSizeCalculation=off
  Lib_MultiBit_Concat2 : Library_DataProcessing_v1/Lib_MultiBit_Concat  SystemSampleTime=-1  VariantActivationTime=update diagram  Latency=0  AutoFrameSizeCalculation=off
  Lib_OutProcessing1 : Library_DataProcessing_v1/Lib_OutProcessing  SystemSampleTime=-1  VariantActivationTime=update diagram  Latency=0  AutoFrameSizeCalculation=off
  Lib_OutProcessing2 : Library_DataProcessing_v1/Lib_OutProcessing  SystemSampleTime=-1  VariantActivationTime=update diagram  Latency=0  AutoFrameSizeCalculation=off
  Mux : Mux  Inputs=8
  OP_ChiefMaster_Battery2_Msg9 : Outport
  wires:
  Bus Selector1/4 -> Data Type Conversion/1  "<IT_sBMS_InternalResistance_BB2_ohms>"
  Bus Selector1/3 -> Mux/7  "<IT_u8BMS_SOC_BB2>"
  Lib_2bytes_Split2/2 -> Mux/6
  Lib_2bytes_Split2/1 -> Mux/5
  Constant1/1 -> Lib_OutProcessing2/2
  Constant3/1 -> Lib_OutProcessing2/3
  Lib_OutProcessing2/1 -> Lib_2bytes_Split2/1
  Bus Selector1/2 -> Lib_OutProcessing2/1  "<IT_sBMS_Current_BB2>"
  Lib_2bytes_Split1/2 -> Mux/4
  Lib_2bytes_Split1/1 -> Mux/3
  Bus Selector1/1 -> Lib_OutProcessing1/1  "<IT_sBMS_VtgInt_BB2>"
  Lib_OutProcessing1/1 -> Lib_2bytes_Split1/1
  Constant2/1 -> Lib_OutProcessing1/3
  Constant/1 -> Lib_OutProcessing1/2
  Lib_MultiBit_Concat2/1 -> Mux/2
  Lib_MultiBit_Concat1/1 -> Mux/1
  Bus Selector6/6 -> Lib_MultiBit_Concat1/8  "<IT_boBMS_SDError_BB2>"
  Bus Selector6/5 -> Extract Bits1/1  "<OT_u8Contactor_FB_State_BB2>"
  Bus Selector6/4 -> Lib_MultiBit_Concat1/5  "<OT_boREQ_HV_ON_BB2>"
  Bus Selector6/3 -> Extract Bits2/1  "<OT_u8ContactorState_BB2>"
  Bus Selector6/2 -> Lib_MultiBit_Concat1/2  "<OT_boREQ_IMD_ON_BB2>"
  Bus Selector6/1 -> Lib_MultiBit_Concat1/1  "<IT_boBMS_Batt2_Availability>"
  OT_Databus/1 -> Bus Selector6/1, Bus Selector1/1, Bus Selector2/1
  Mux/1 -> OP_ChiefMaster_Battery2_Msg9/1
  Data Type Conversion/1 -> Mux/8
  Extract Bits1/1 -> Lib_MultiBit_Concat1/6
  Extract Bits2/1 -> Lib_MultiBit_Concat1/3
  Constant4/1 -> Lib_MultiBit_Concat1/4, Lib_MultiBit_Concat1/7
  Bus Selector2/1 -> Lib_MultiBit_Concat2/1  "<IT_boBMS_HV_REL_ON_BB2>"
  Bus Selector2/2 -> Lib_MultiBit_Concat2/2  "<IT_boBMS_HV_Minus_Sense_BB2>"
  Bus Selector2/3 -> Lib_MultiBit_Concat2/3  "<IT_boBMS_HV_Plus_Sense_BB2>"
  Bus Selector2/4 -> Lib_MultiBit_Concat2/4  "<IT_boBMS_InsulationReadyOK_B2>"
  Bus Selector2/5 -> Lib_MultiBit_Concat2/5  "<IT_boBMS_InsulationSDError_B2>"
  Bus Selector2/6 -> Lib_MultiBit_Concat2/6  "<IT_boBMS_IMD_Active_BB2>"
  Bus Selector2/7 -> Lib_MultiBit_Concat2/7  "<IT_boBMS_Error_BB2>"
  Bus Selector2/8 -> Lib_MultiBit_Concat2/8  "<IT_boBMS_Warning_BB2>"

== system ChiefMaster_TTC580/ChiefMaster/Output Processing/CM_OBD/CM_Battery2_Msg11 ==
  OT_Databus : Inport
  Bus Selector1 : BusSelector  OutputSignals=FL_Databus.IT_Databus.IT_BatterySignal_Databus.IT_sBMS_ChargeCurrentPrognosis_BB2,FL_Databus.IT_Databus.IT_BatterySignal_Databus.IT_sBMS_DisChargeCurrentPrognosis_BB2,FL_Databus.IT_Databus.IT_BatterySignal_Databus.IT_sBMS_InsulationResistance_BB2,FL_Databus.IT_Databus.IT_BatterySignal_Databus.IT_boBMS_InsulationResistance_Minus_kOhm_BB2
  Constant{1..2,5,7} (4 alike) : Constant  Value=0  OutDataTypeStr=single
  Constant3 : Constant  Value=0.1  OutDataTypeStr=single
  Constant4 : Constant  Value=0.1  OutDataTypeStr=single
  Constant6 : Constant  Value=100  OutDataTypeStr=single
  Constant8 : Constant  Value=100  OutDataTypeStr=single
  Lib_2bytes_Split{1..4} (4 alike) : Library_DataProcessing_v1/Lib_2bytes_Split  SystemSampleTime=-1  VariantActivationTime=update diagram  Latency=0  AutoFrameSizeCalculation=off
  Lib_OutProcessing{1..4} (4 alike) : Library_DataProcessing_v1/Lib_OutProcessing  SystemSampleTime=-1  VariantActivationTime=update diagram  Latency=0  AutoFrameSizeCalculation=off
  Mux : Mux  Inputs=8
  OP_ChiefMaster_Battery2_Msg10 : Outport
  wires:
  Lib_2bytes_Split4/2 -> Mux/8
  Lib_2bytes_Split4/1 -> Mux/7
  Constant8/1 -> Lib_OutProcessing4/3
  Lib_OutProcessing4/1 -> Lib_2bytes_Split4/1
  Constant7/1 -> Lib_OutProcessing4/2
  Lib_2bytes_Split3/2 -> Mux/6
  Lib_2bytes_Split3/1 -> Mux/5
  Constant5/1 -> Lib_OutProcessing3/2
  Lib_OutProcessing3/1 -> Lib_2bytes_Split3/1
  Constant6/1 -> Lib_OutProcessing3/3
  Lib_2bytes_Split1/2 -> Mux/4
  Lib_2bytes_Split1/1 -> Mux/3
  Constant4/1 -> Lib_OutProcessing1/3
  Lib_OutProcessing1/1 -> Lib_2bytes_Split1/1
  Constant2/1 -> Lib_OutProcessing1/2
  Lib_2bytes_Split2/2 -> Mux/2
  Lib_2bytes_Split2/1 -> Mux/1
  Constant1/1 -> Lib_OutProcessing2/2
  Lib_OutProcessing2/1 -> Lib_2bytes_Split2/1
  Constant3/1 -> Lib_OutProcessing2/3
  Bus Selector1/4 -> Lib_OutProcessing4/1  "<IT_boBMS_InsulationResistance_Minus_kOhm_BB2>"
  Bus Selector1/3 -> Lib_OutProcessing3/1  "<IT_sBMS_InsulationResistance_BB2>"
  Bus Selector1/2 -> Lib_OutProcessing1/1  "<IT_sBMS_DisChargeCurrentPrognosis_BB2>"
  Bus Selector1/1 -> Lib_OutProcessing2/1  "<IT_sBMS_ChargeCurrentPrognosis_BB2>"
  Mux/1 -> OP_ChiefMaster_Battery2_Msg10/1
  OT_Databus/1 -> Bus Selector1/1

== system ChiefMaster_TTC580/ChiefMaster/Output Processing/CM_OBD/CM_Battery2_Msg12 ==
  OT_Databus : Inport
  Bus Selector1 : BusSelector  OutputSignals=FL_Databus.IT_Databus.IT_BatterySignal_Databus.IP_sBMS_MinTemp_degC_BB2,FL_Databus.IT_Databus.IT_BatterySignal_Databus.IP_sBMS_MaxTemp_degC_BB2,FL_Databus.IT_Databus.IT_BatterySignal_Databus.IP_sBMS_MinCellVoltage_BB2,FL_Databus.IT_Databus.IT_BatterySignal_Databus.IP_sBMS_MaxCellVoltage_BB2
  Constant1 : Constant  Value=-40  OutDataTypeStr=single
  Constant2 : Constant  Value=-40  OutDataTypeStr=single
  Constant3 : Constant  OutDataTypeStr=single
  Constant4 : Constant  OutDataTypeStr=single
  Constant5 : Constant  Value=0  OutDataTypeStr=single
  Constant6 : Constant  Value=0.1  OutDataTypeStr=single
  Constant7 : Constant  Value=0  OutDataTypeStr=single
  Constant8 : Constant  Value=0.1  OutDataTypeStr=single
  Constant9 : Constant  Value=0  OutDataTypeStr=uint8
  Data Type Conversion : DataTypeConversion  OutDataTypeStr=uint8  SaturateOnIntegerOverflow=off  RndMeth=Floor
  Data Type Conversion1 : DataTypeConversion  OutDataTypeStr=uint8  SaturateOnIntegerOverflow=off  RndMeth=Floor
  Lib_2bytes_Split3 : Library_DataProcessing_v1/Lib_2bytes_Split  SystemSampleTime=-1  VariantActivationTime=update diagram  Latency=0  AutoFrameSizeCalculation=off
  Lib_2bytes_Split4 : Library_DataProcessing_v1/Lib_2bytes_Split  SystemSampleTime=-1  VariantActivationTime=update diagram  Latency=0  AutoFrameSizeCalculation=off
  Lib_OutProcessing{1..4} (4 alike) : Library_DataProcessing_v1/Lib_OutProcessing  SystemSampleTime=-1  VariantActivationTime=update diagram  Latency=0  AutoFrameSizeCalculation=off
  Mux : Mux  Inputs=8
  OP_ChiefMaster_Battery1_Msg8 : Outport
  wires:
  OT_Databus/1 -> Bus Selector1/1
  Mux/1 -> OP_ChiefMaster_Battery1_Msg8/1
  Bus Selector1/1 -> Lib_OutProcessing2/1  "<IP_sBMS_MinTemp_degC_BB2>"
  Bus Selector1/2 -> Lib_OutProcessing1/1  "<IP_sBMS_MaxTemp_degC_BB2>"
  Bus Selector1/3 -> Lib_OutProcessing3/1  "<IP_sBMS_MinCellVoltage_BB2>"
  Bus Selector1/4 -> Lib_OutProcessing4/1  "<IP_sBMS_MaxCellVoltage_BB2>"
  Constant3/1 -> Lib_OutProcessing2/3
  Lib_OutProcessing2/1 -> Data Type Conversion/1
  Constant1/1 -> Lib_OutProcessing2/2
  Constant2/1 -> Lib_OutProcessing1/2
  Lib_OutProcessing1/1 -> Data Type Conversion1/1
  Constant4/1 -> Lib_OutProcessing1/3
  Constant6/1 -> Lib_OutProcessing3/3
  Lib_OutProcessing3/1 -> Lib_2bytes_Split3/1
  Constant5/1 -> Lib_OutProcessing3/2
  Constant7/1 -> Lib_OutProcessing4/2
  Lib_OutProcessing4/1 -> Lib_2bytes_Split4/1
  Constant8/1 -> Lib_OutProcessing4/3
  Constant9/1 -> Mux/8, Mux/7
  Data Type Conversion/1 -> Mux/1
  Data Type Conversion1/1 -> Mux/2
  Lib_2bytes_Split3/1 -> Mux/3
  Lib_2bytes_Split3/2 -> Mux/4
  Lib_2bytes_Split4/1 -> Mux/5
  Lib_2bytes_Split4/2 -> Mux/6

== system ChiefMaster_TTC580/ChiefMaster/Output Processing/CM_OBD/CM_Battery3_Msg13 ==
  OT_Databus : Inport
  Bus Selector1 : BusSelector  OutputSignals=FL_Databus.IT_Databus.IT_BatterySignal_Databus.IT_sBMS_VtgInt_BB3,FL_Databus.IT_Databus.IT_BatterySignal_Databus.IT_sBMS_Current_BB3,FL_Databus.IT_Databus.IT_BatterySignal_Databus.IT_u8BMS_SOC_BB3,FL_Databus.IT_Databus.IT_BatterySignal_Databus.IT_sBMS_InternalResistance_BB3_ohms
  Bus Selector2 : BusSelector  OutputSignals=FL_Databus.IT_Databus.IT_BatterySignal_Databus.IT_boBMS_HV_REL_ON_BB3,FL_Databus.IT_Databus.IT_BatterySignal_Databus.IT_boBMS_HV_Minus_Sense_BB3,FL_Databus.IT_Databus.IT_BatterySignal_Databus.IT_boBMS_HV_Plus_Sense_BB3,FL_Databus.IT_Databus.IT_BatterySignal_Databus.IT_boBMS_InsulationReadyOK_B3,FL_Databus.IT_Databus.IT_BatterySignal_Databus.IT_boBMS_InsulationSDError_B3,FL_Databus.IT_Databus.IT_BatterySignal_Databus.IT_boBMS_IMD_Active_BB3,FL_Databus.IT_Databus.IT_BatterySignal_Databus.IT_boBMS_Error_BB3,FL_Databus.IT_Databus.IT_BatterySignal_Databus.IT_boBMS_Warning_BB3
  Bus Selector6 : BusSelector  OutputSignals=FL_Databus.IT_Databus.IT_BatterySignal_Databus.IT_boBMS_Batt3_Availability,OT_IMD_Databus.OT_boREQ_IMD_ON_BB3,OT_BatteryBox_HVControl_Databus.OT_u8ContactorState_BB3,OT_BatteryBox_HVControl_Databus.OT_boREQ_HV_ON_BB3,OT_BatteryBox_HVControl_Databus.OT_u8Contactor_FB_State_BB3,FL_Databus.IT_Databus.IT_BatterySignal_Databus.IT_boBMS_SDError_BB3
  Constant : Constant  Value=0  OutDataTypeStr=single
  Constant1 : Constant  Value=0  OutDataTypeStr=single
  Constant2 : Constant  Value=0.1  OutDataTypeStr=single
  Constant3 : Constant  Value=0.1  OutDataTypeStr=single
  Constant4 : Constant  Value=0  OutDataTypeStr=uint8
  Data Type Conversion1 : DataTypeConversion  OutDataTypeStr=uint8  SaturateOnIntegerOverflow=off  RndMeth=Floor
  Extract Bits1 : simulink/Logic and Bit Operations/Extract Bits  bitsToExtract=Range of bits  numBits=8  bitIdxRange=[0 1]  outScalingMode=Preserve fixed-point scaling
  Extract Bits2 : simulink/Logic and Bit Operations/Extract Bits  bitsToExtract=Range of bits  numBits=8  bitIdxRange=[0 1]  outScalingMode=Preserve fixed-point scaling
  Lib_2bytes_Split1 : Library_DataProcessing_v1/Lib_2bytes_Split  SystemSampleTime=-1  VariantActivationTime=update diagram  Latency=0  AutoFrameSizeCalculation=off
  Lib_2bytes_Split2 : Library_DataProcessing_v1/Lib_2bytes_Split  SystemSampleTime=-1  VariantActivationTime=update diagram  Latency=0  AutoFrameSizeCalculation=off
  Lib_MultiBit_Concat10 : Library_DataProcessing_v1/Lib_MultiBit_Concat  SystemSampleTime=-1  VariantActivationTime=update diagram  Latency=0  AutoFrameSizeCalculation=off
  Lib_MultiBit_Concat7 : Library_DataProcessing_v1/Lib_MultiBit_Concat  SystemSampleTime=-1  VariantActivationTime=update diagram  Latency=0  AutoFrameSizeCalculation=off
  Lib_OutProcessing1 : Library_DataProcessing_v1/Lib_OutProcessing  SystemSampleTime=-1  VariantActivationTime=update diagram  Latency=0  AutoFrameSizeCalculation=off
  Lib_OutProcessing2 : Library_DataProcessing_v1/Lib_OutProcessing  SystemSampleTime=-1  VariantActivationTime=update diagram  Latency=0  AutoFrameSizeCalculation=off
  Mux : Mux  Inputs=8
  OP_ChiefMaster_Battery3_Msg11 : Outport
  wires:
  Mux/1 -> OP_ChiefMaster_Battery3_Msg11/1
  OT_Databus/1 -> Bus Selector1/1, Bus Selector2/1, Bus Selector6/1
  Lib_MultiBit_Concat7/1 -> Mux/1
  Lib_MultiBit_Concat10/1 -> Mux/2
  Constant/1 -> Lib_OutProcessing1/2
  Constant2/1 -> Lib_OutProcessing1/3
  Lib_OutProcessing1/1 -> Lib_2bytes_Split1/1
  Bus Selector1/1 -> Lib_OutProcessing1/1  "<IT_sBMS_VtgInt_BB3>"
  Lib_2bytes_Split1/1 -> Mux/3
  Lib_2bytes_Split1/2 -> Mux/4
  Bus Selector1/2 -> Lib_OutProcessing2/1  "<IT_sBMS_Current_BB3>"
  Lib_OutProcessing2/1 -> Lib_2bytes_Split2/1
  Constant3/1 -> Lib_OutProcessing2/3
  Constant1/1 -> Lib_OutProcessing2/2
  Lib_2bytes_Split2/1 -> Mux/5
  Lib_2bytes_Split2/2 -> Mux/6
  Bus Selector1/3 -> Mux/7  "<IT_u8BMS_SOC_BB3>"
  Bus Selector1/4 -> Data Type Conversion1/1  "<IT_sBMS_InternalResistance_BB3_ohms>"
  Data Type Conversion1/1 -> Mux/8
  Extract Bits2/1 -> Lib_MultiBit_Concat7/3
  Bus Selector2/1 -> Lib_MultiBit_Concat10/1  "<IT_boBMS_HV_REL_ON_BB3>"
  Bus Selector2/2 -> Lib_MultiBit_Concat10/2  "<IT_boBMS_HV_Minus_Sense_BB3>"
  Bus Selector2/3 -> Lib_MultiBit_Concat10/3  "<IT_boBMS_HV_Plus_Sense_BB3>"
  Bus Selector2/4 -> Lib_MultiBit_Concat10/4  "<IT_boBMS_InsulationReadyOK_B3>"
  Bus Selector2/5 -> Lib_MultiBit_Concat10/5  "<IT_boBMS_InsulationSDError_B3>"
  Bus Selector2/6 -> Lib_MultiBit_Concat10/6  "<IT_boBMS_IMD_Active_BB3>"
  Bus Selector2/7 -> Lib_MultiBit_Concat10/7  "<IT_boBMS_Error_BB3>"
  Bus Selector2/8 -> Lib_MultiBit_Concat10/8  "<IT_boBMS_Warning_BB3>"
  Bus Selector6/1 -> Lib_MultiBit_Concat7/1  "<IT_boBMS_Batt3_Availability>"
  Bus Selector6/2 -> Lib_MultiBit_Concat7/2  "<OT_boREQ_IMD_ON_BB3>"
  Bus Selector6/3 -> Extract Bits2/1  "<OT_u8ContactorState_BB3>"
  Bus Selector6/4 -> Lib_MultiBit_Concat7/5  "<OT_boREQ_HV_ON_BB3>"
  Constant4/1 -> Lib_MultiBit_Concat7/7, Lib_MultiBit_Concat7/4
  Bus Selector6/5 -> Extract Bits1/1  "<OT_u8Contactor_FB_State_BB3>"
  Extract Bits1/1 -> Lib_MultiBit_Concat7/6
  Bus Selector6/6 -> Lib_MultiBit_Concat7/8  "<IT_boBMS_SDError_BB3>"

== system ChiefMaster_TTC580/ChiefMaster/Output Processing/CM_OBD/CM_Battery3_Msg14 ==
  OT_Databus : Inport
  Bus Selector1 : BusSelector  OutputSignals=FL_Databus.IT_Databus.IT_BatterySignal_Databus.IT_sBMS_ChargeCurrentPrognosis_BB3,FL_Databus.IT_Databus.IT_BatterySignal_Databus.IT_sBMS_DisChargeCurrentPrognosis_BB3,FL_Databus.IT_Databus.IT_BatterySignal_Databus.IT_sBMS_InsulationResistance_BB3,FL_Databus.IT_Databus.IT_BatterySignal_Databus.IT_boBMS_InsulationResistance_Minus_kOhm_BB3
  Constant{1..2,5,7} (4 alike) : Constant  Value=0  OutDataTypeStr=single
  Constant3 : Constant  Value=0.1  OutDataTypeStr=single
  Constant4 : Constant  Value=0.1  OutDataTypeStr=single
  Constant6 : Constant  Value=100  OutDataTypeStr=single
  Constant8 : Constant  Value=100  OutDataTypeStr=single
  Lib_2bytes_Split{1..4} (4 alike) : Library_DataProcessing_v1/Lib_2bytes_Split  SystemSampleTime=-1  VariantActivationTime=update diagram  Latency=0  AutoFrameSizeCalculation=off
  Lib_OutProcessing{1..4} (4 alike) : Library_DataProcessing_v1/Lib_OutProcessing  SystemSampleTime=-1  VariantActivationTime=update diagram  Latency=0  AutoFrameSizeCalculation=off
  Mux : Mux  Inputs=8
  OP_ChiefMaster_Battery3_Msg12 : Outport
  wires:
  OT_Databus/1 -> Bus Selector1/1
  Mux/1 -> OP_ChiefMaster_Battery3_Msg12/1
  Bus Selector1/1 -> Lib_OutProcessing2/1  "<IT_sBMS_ChargeCurrentPrognosis_BB3>"
  Bus Selector1/2 -> Lib_OutProcessing1/1  "<IT_sBMS_DisChargeCurrentPrognosis_BB3>"
  Bus Selector1/3 -> Lib_OutProcessing3/1  "<IT_sBMS_InsulationResistance_BB3>"
  Bus Selector1/4 -> Lib_OutProcessing4/1  "<IT_boBMS_InsulationResistance_Minus_kOhm_BB3>"
  Constant3/1 -> Lib_OutProcessing2/3
  Lib_OutProcessing2/1 -> Lib_2bytes_Split2/1
  Constant1/1 -> Lib_OutProcessing2/2
  Lib_2bytes_Split2/1 -> Mux/1
  Lib_2bytes_Split2/2 -> Mux/2
  Constant2/1 -> Lib_OutProcessing1/2
  Lib_OutProcessing1/1 -> Lib_2bytes_Split1/1
  Constant4/1 -> Lib_OutProcessing1/3
  Lib_2bytes_Split1/1 -> Mux/3
  Lib_2bytes_Split1/2 -> Mux/4
  Constant6/1 -> Lib_OutProcessing3/3
  Lib_OutProcessing3/1 -> Lib_2bytes_Split3/1
  Constant5/1 -> Lib_OutProcessing3/2
  Lib_2bytes_Split3/1 -> Mux/5
  Lib_2bytes_Split3/2 -> Mux/6
  Constant7/1 -> Lib_OutProcessing4/2
  Lib_OutProcessing4/1 -> Lib_2bytes_Split4/1
  Constant8/1 -> Lib_OutProcessing4/3
  Lib_2bytes_Split4/1 -> Mux/7
  Lib_2bytes_Split4/2 -> Mux/8

== system ChiefMaster_TTC580/ChiefMaster/Output Processing/CM_OBD/CM_Battery3_Msg15 ==
  OT_Databus : Inport
  Bus Selector1 : BusSelector  OutputSignals=FL_Databus.IT_Databus.IT_BatterySignal_Databus.IP_sBMS_MinTemp_degC_BB3,FL_Databus.IT_Databus.IT_BatterySignal_Databus.IP_sBMS_MaxTemp_degC_BB3,FL_Databus.IT_Databus.IT_BatterySignal_Databus.IP_sBMS_MinCellVoltage_BB3,FL_Databus.IT_Databus.IT_BatterySignal_Databus.IP_sBMS_MaxCellVoltage_BB3
  Constant1 : Constant  Value=-40  OutDataTypeStr=single
  Constant2 : Constant  Value=-40  OutDataTypeStr=single
  Constant3 : Constant  OutDataTypeStr=single
  Constant4 : Constant  OutDataTypeStr=single
  Constant5 : Constant  Value=0  OutDataTypeStr=single
  Constant6 : Constant  Value=0.1  OutDataTypeStr=single
  Constant7 : Constant  Value=0  OutDataTypeStr=single
  Constant8 : Constant  Value=0.1  OutDataTypeStr=single
  Constant9 : Constant  Value=0  OutDataTypeStr=uint8
  Data Type Conversion : DataTypeConversion  OutDataTypeStr=uint8  SaturateOnIntegerOverflow=off  RndMeth=Floor
  Data Type Conversion1 : DataTypeConversion  OutDataTypeStr=uint8  SaturateOnIntegerOverflow=off  RndMeth=Floor
  Lib_2bytes_Split3 : Library_DataProcessing_v1/Lib_2bytes_Split  SystemSampleTime=-1  VariantActivationTime=update diagram  Latency=0  AutoFrameSizeCalculation=off
  Lib_2bytes_Split4 : Library_DataProcessing_v1/Lib_2bytes_Split  SystemSampleTime=-1  VariantActivationTime=update diagram  Latency=0  AutoFrameSizeCalculation=off
  Lib_OutProcessing{1..4} (4 alike) : Library_DataProcessing_v1/Lib_OutProcessing  SystemSampleTime=-1  VariantActivationTime=update diagram  Latency=0  AutoFrameSizeCalculation=off
  Mux : Mux  Inputs=8
  OP_ChiefMaster_Battery1_Msg8 : Outport
  wires:
  Constant8/1 -> Lib_OutProcessing4/3
  Lib_OutProcessing4/1 -> Lib_2bytes_Split4/1
  Constant7/1 -> Lib_OutProcessing4/2
  Constant5/1 -> Lib_OutProcessing3/2
  Lib_OutProcessing3/1 -> Lib_2bytes_Split3/1
  Constant6/1 -> Lib_OutProcessing3/3
  Constant4/1 -> Lib_OutProcessing1/3
  Lib_OutProcessing1/1 -> Data Type Conversion/1
  Constant2/1 -> Lib_OutProcessing1/2
  Lib_OutProcessing2/1 -> Data Type Conversion1/1
  Constant1/1 -> Lib_OutProcessing2/2
  Constant3/1 -> Lib_OutProcessing2/3
  Bus Selector1/4 -> Lib_OutProcessing4/1  "<IP_sBMS_MaxCellVoltage_BB3>"
  Bus Selector1/3 -> Lib_OutProcessing3/1  "<IP_sBMS_MinCellVoltage_BB3>"
  Bus Selector1/2 -> Lib_OutProcessing1/1  "<IP_sBMS_MaxTemp_degC_BB3>"
  Bus Selector1/1 -> Lib_OutProcessing2/1  "<IP_sBMS_MinTemp_degC_BB3>"
  Mux/1 -> OP_ChiefMaster_Battery1_Msg8/1
  OT_Databus/1 -> Bus Selector1/1
  Lib_2bytes_Split3/1 -> Mux/3
  Lib_2bytes_Split3/2 -> Mux/4
  Lib_2bytes_Split4/1 -> Mux/5
  Lib_2bytes_Split4/2 -> Mux/6
  Constant9/1 -> Mux/7, Mux/8
  Data Type Conversion/1 -> Mux/2
  Data Type Conversion1/1 -> Mux/1

== system ChiefMaster_TTC580/ChiefMaster/Output Processing/CM_OBD/CM_IP_Msg1 ==
  OT_Databus : Inport
  Bus Selector6 : BusSelector  OutputSignals=FL_Databus.IT_Databus.IT_HW_Input_Databus.IT_boHW_KL15,FL_Databus.IT_Databus.IT_UDC_Databus.IT_boUDC_KL15_D,FL_Databus.IT_Databus.IT_UDC_Databus.IT_boUDC_KL15_C,FL_Databus.IT_Databus.IT_HW_Input_Databus.IT_boHW_HVIL_BDU,FL_Databus.IT_Databus.IT_HW_Input_Databus.IT_boHW_HVIL_Components,FL_Databus.IT_Databus.IT_HW_Input_Databus.IT_boHW_HVIL_Battery,FL_Databus.IT_Databus.IT_HW_Input_Databus.IT_boHW_MainHV_Plus_FB,FL_Databus.IT_Databus.IT_HW_Input_Databus.IT_boHW_MainHV_Minus_FB,FL_Databus.IT_Databus.IT_HW_Input_Databus.IT_sHW_EmergencyButton_NC,FL_Databus.IT_Databus.IT_HW_Input_Databus.IT_boHW_EmergencyButton_NO,FL_Databus.IT_Databus.IT_HW_Input_Databus.IT_boHW_ResetButton_LED_NO,FL_Databus.IT_Databus.IT_HW_Input_Databus.IT_boHW_Proximity_BB1,FL_Databus.IT_Databus.IT_HW_Input_Databus.IT_boHW_Proximity_BB2,FL_Databus.IT_Databus.IT_HW_Input_Databus.IT_boHW_Proximity_BB3,FL_Databus.IT_Databus.IT_HW_Input_Databus.IT_boHW_DCHV_Plus_FB,FL_Databus.IT_Databus.IT_HW_Input_Databus.IT_boHW_DCHV_Minus_FB,FL_Databus.IT_Databus.IT_SelectBattery_Databus.IT_u8Select_Battery1,FL_Databus.IT_Databus.IT_SelectBattery_Databus.IT_u8Select_Battery2,FL_Databus.IT_Databus.IT_SelectBattery_Databus.IT_u8Select_Battery3,FL_Databus.IT_Databus.IT_UDC_Databus.IT_boUDC_SafeToShutdown,FL_Databus.IT_Databus.IT_HW_Input_Databus.IT_boHW_HVIL_Overrule,FL_Databus.IT_Databus.IT_UDC_Databus.IT_sUDC_LoadVoltage_V
  Constant : Constant  Value=0  OutDataTypeStr=uint8
  Constant1 : Constant  Value=0  OutDataTypeStr=uint8
  Extract Bits : simulink/Logic and Bit Operations/Extract Bits  bitsToExtract=Range of bits  numBits=8  bitIdxRange=[0 1]  outScalingMode=Preserve fixed-point scaling
  Extract Bits1 : simulink/Logic and Bit Operations/Extract Bits  bitsToExtract=Range of bits  numBits=8  bitIdxRange=[0 1]  outScalingMode=Preserve fixed-point scaling
  Extract Bits2 : simulink/Logic and Bit Operations/Extract Bits  bitsToExtract=Range of bits  numBits=8  bitIdxRange=[0 1]  outScalingMode=Preserve fixed-point scaling
  Lib_MultiBit_Concat1 : Library_DataProcessing_v1/Lib_MultiBit_Concat  SystemSampleTime=-1  VariantActivationTime=update diagram  Latency=0  AutoFrameSizeCalculation=off
  Lib_MultiBit_Concat10 : Library_DataProcessing_v1/Lib_MultiBit_Concat  SystemSampleTime=-1  VariantActivationTime=update diagram  Latency=0  AutoFrameSizeCalculation=off
  Lib_MultiBit_Concat7 : Library_DataProcessing_v1/Lib_MultiBit_Concat  SystemSampleTime=-1  VariantActivationTime=update diagram  Latency=0  AutoFrameSizeCalculation=off
  LoadVoltage : Subsystem
  Mux : Mux  Inputs=8
  OP_ChiefMaster_IP_Msg1 : Outport
  wires:
  Lib_MultiBit_Concat10/1 -> Mux/2
  Lib_MultiBit_Concat7/1 -> Mux/1
  Bus Selector6/16 -> Lib_MultiBit_Concat10/8  "<IT_boHW_DCHV_Minus_FB>"
  Bus Selector6/15 -> Lib_MultiBit_Concat10/7  "<IT_boHW_DCHV_Plus_FB>"
  Bus Selector6/14 -> Lib_MultiBit_Concat10/6  "<IT_boHW_Proximity_BB3>"
  Bus Selector6/13 -> Lib_MultiBit_Concat10/5  "<IT_boHW_Proximity_BB2>"
  Bus Selector6/12 -> Lib_MultiBit_Concat10/4  "<IT_boHW_Proximity_BB1>"
  Bus Selector6/11 -> Lib_MultiBit_Concat10/3  "<IT_boHW_ResetButton_LED_NO>"
  Bus Selector6/10 -> Lib_MultiBit_Concat10/2  "<IT_boHW_EmergencyButton_NO>"
  Bus Selector6/9 -> Lib_MultiBit_Concat10/1  "<IT_sHW_EmergencyButton_NC>"
  Bus Selector6/8 -> Lib_MultiBit_Concat7/8  "<IT_boHW_MainHV_Minus_FB>"
  Bus Selector6/7 -> Lib_MultiBit_Concat7/7  "<IT_boHW_MainHV_Plus_FB>"
  Bus Selector6/6 -> Lib_MultiBit_Concat7/6  "<IT_boHW_HVIL_Battery>"
  Bus Selector6/5 -> Lib_MultiBit_Concat7/5  "<IT_boHW_HVIL_Components>"
  Bus Selector6/4 -> Lib_MultiBit_Concat7/4  "<IT_boHW_HVIL_BDU>"
  Bus Selector6/3 -> Lib_MultiBit_Concat7/3  "<IT_boUDC_KL15_C>"
  Bus Selector6/2 -> Lib_MultiBit_Concat7/2  "<IT_boUDC_KL15_D>"
  Bus Selector6/1 -> Lib_MultiBit_Concat7/1  "<IT_boHW_KL15>"
  OT_Databus/1 -> Bus Selector6/1
  Bus Selector6/17 -> Extract Bits2/1  "<IT_u8Select_Battery1>"
  Bus Selector6/18 -> Extract Bits/1  "<IT_u8Select_Battery2>"
  Bus Selector6/19 -> Extract Bits1/1  "<IT_u8Select_Battery3>"
  Bus Selector6/20 -> Lib_MultiBit_Concat1/7  "<IT_boUDC_SafeToShutdown>"
  Bus Selector6/22 -> LoadVoltage/1(LoadVoltage)  "<IT_sUDC_LoadVoltage_V>"
  Lib_MultiBit_Concat1/1 -> Mux/3
  Constant/1 -> Lib_MultiBit_Concat1/6, Lib_MultiBit_Concat1/2, Lib_MultiBit_Concat1/4
  LoadVoltage/1(u8byte_LSB) -> Mux/4
  LoadVoltage/2(u8byte_MSB) -> Mux/5
  Extract Bits/1 -> Lib_MultiBit_Concat1/3
  Extract Bits2/1 -> Lib_MultiBit_Concat1/1
  Extract Bits1/1 -> Lib_MultiBit_Concat1/5
  Constant1/1 -> Mux/8, Mux/7, Mux/6
  Mux/1 -> OP_ChiefMaster_IP_Msg1/1
  Bus Selector6/21 -> Lib_MultiBit_Concat1/8  "<IT_boHW_HVIL_Overrule>"
